simulink model "SrmAmLinearApcMmk1"  (R2013b)
settings: Solver=ode45  StartTime=0.0  StopTime=10.0  RelTol=1e-3
settings Model: Creator=mamingkai  LastModifiedBy=mamingkai

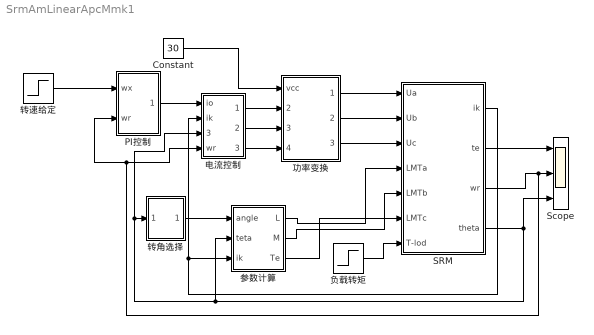
== system SrmAmLinearApcMmk1 ==
  Constant : Constant  Value=30
  PI控制 : Subsystem
  SRM : Subsystem
  Scope : Scope  NumInputPorts=3
      settings: YMin=-5~-5~-5  YMax=5~5~5
  功率变换 : Subsystem
  参数计算 : Subsystem
  电流控制 : Subsystem
  负载转矩 : Step  SampleTime=0
  转角选择 : Subsystem
  转速给定 : Step  SampleTime=0
  wires:
  转速给定/1 -> PI控制/1(wx)
  电流控制/1(Out1) -> 功率变换/2(PUSEA)
  电流控制/2(Out2) -> 功率变换/3(PUDEB)
  电流控制/3(Out3) -> 功率变换/4(PUSEC)
  PI控制/1(Out1) -> 电流控制/1(io)
  Constant/1 -> 功率变换/1(vcc)
  功率变换/1(Out1) -> SRM/1(Ua)
  功率变换/2(Out2) -> SRM/2(Ub)
  功率变换/3(Out3) -> SRM/3(Uc)
  转角选择/1(Out1) -> 参数计算/1(angle)
  SRM/1(ik) -> 参数计算/3(ik), 电流控制/2(ik)
  SRM/3(wr) -> PI控制/2(wr), 电流控制/4(wr), Scope/2
  SRM/4(theta) -> Scope/3, 转角选择/1(In1), 电流控制/3(teta), 参数计算/2(teta)
  SRM/2(te) -> Scope/1
  参数计算/1(L) -> SRM/4(LMTa)
  参数计算/2(M) -> SRM/5(LMTb)
  参数计算/3(Te) -> SRM/6(LMTc)
  负载转矩/1 -> SRM/7(T-lod)

== system SrmAmLinearApcMmk1/PI控制 ==
  wx : Inport
  wr : Inport  Port=2
  Gain : Gain
  Gain1 : Gain
  Integrator : Integrator
  Saturation : Saturate
  netsum : Sum  Inputs=2  SaturateOnIntegerOverflow=on  InputSameDT=on  OutDataTypeStr=Inherit: Same as first input
  netsum1 : Sum  Inputs=+-  SaturateOnIntegerOverflow=on  InputSameDT=on  OutDataTypeStr=Inherit: Same as first input
  Out1 : Outport
  wires:
  wx/1 -> netsum1/1
  wr/1 -> netsum1/2
  netsum1/1 -> Gain/1, Gain1/1
  Gain1/1 -> Integrator/1
  Integrator/1 -> netsum/2
  Gain/1 -> netsum/1
  netsum/1 -> Saturation/1
  Saturation/1 -> Out1/1

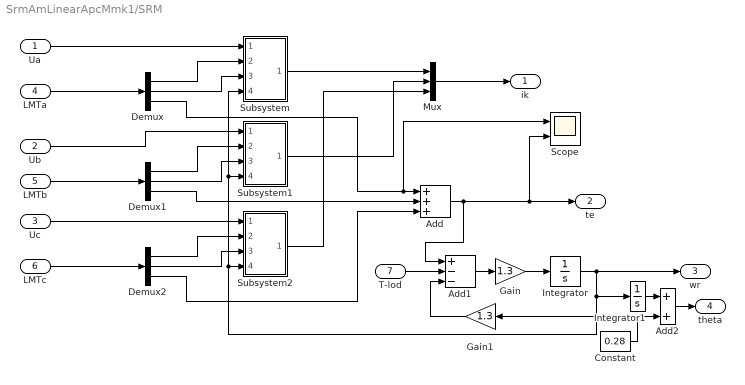
== system SrmAmLinearApcMmk1/SRM ==
  Ua : Inport
  Ub : Inport  Port=2
  Uc : Inport  Port=3
  LMTa : Inport  Port=4
  LMTb : Inport  Port=5
  LMTc : Inport  Port=6
  T-lod : Inport  Port=7
  Add : Sum  Inputs=+++
  Add1 : Sum  Inputs=+--
  Add2 : Sum
  Constant : Constant  Value=0.28
  Demux : Demux  Outputs=3
  Demux1 : Demux  Outputs=3
  Demux2 : Demux  Outputs=3
  Gain : Gain  Gain=1.3
  Gain1 : Gain  Gain=1.3
  Integrator : Integrator
  Integrator1 : Integrator
  Mux : Mux  Inputs=3
  Scope : Scope  NumInputPorts=2
      settings: YMin=-5~-5  YMax=5~5
  Subsystem : Subsystem
  Subsystem1 : Subsystem
  Subsystem2 : Subsystem
  ik : Outport
  te : Outport  Port=2
  wr : Outport  Port=3
  theta : Outport  Port=4
  wires:
  LMTa/1 -> Demux/1
  Demux/1 -> Subsystem/2(In2)
  Demux/2 -> Subsystem/3(In3)
  Demux/3 -> Scope/1, Add/1
  Ub/1 -> Subsystem1/1(In1)
  Demux1/1 -> Subsystem1/2(In2)
  Demux1/2 -> Subsystem1/3(In3)
  Demux1/3 -> Add/2
  Uc/1 -> Subsystem2/1(In1)
  LMTc/1 -> Demux2/1
  LMTb/1 -> Demux1/1
  Demux2/1 -> Subsystem2/2(In2)
  Demux2/2 -> Subsystem2/3(In3)
  Demux2/3 -> Add/3
  Integrator/1 -> wr/1, Subsystem2/4(In4), Subsystem1/4(In4), Subsystem/4(In4), Gain1/1, Integrator1/1
  Subsystem/1(Out1) -> Mux/1
  Subsystem1/1(Out1) -> Mux/2
  Subsystem2/1(Out1) -> Mux/3
  Mux/1 -> ik/1
  Add/1 -> te/1, Scope/2, Add1/1
  T-lod/1 -> Add1/2
  Gain1/1 -> Add1/3
  Add1/1 -> Gain/1
  Gain/1 -> Integrator/1
  Add2/1 -> theta/1
  Integrator1/1 -> Add2/1
  Constant/1 -> Add2/2
  Ua/1 -> Subsystem/1(In1)

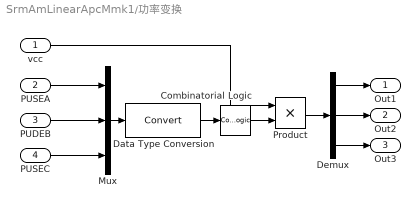
== system SrmAmLinearApcMmk1/功率变换 ==
  vcc : Inport
  PUSEA : Inport  Port=2
  PUDEB : Inport  Port=3
  PUSEC : Inport  Port=4
  Combinatorial Logic : CombinatorialLogic
  Data Type Conversion : DataTypeConversion
  Demux : Demux  Outputs=3
  Mux : Mux  Inputs=3
  Product : Product
  Out1 : Outport
  Out2 : Outport  Port=2
  Out3 : Outport  Port=3
  wires:
  PUSEA/1 -> Mux/1
  Demux/1 -> Out1/1
  Product/1 -> Demux/1
  Demux/2 -> Out2/1
  Demux/3 -> Out3/1
  PUDEB/1 -> Mux/2
  PUSEC/1 -> Mux/3
  Combinatorial Logic/1 -> Product/2
  vcc/1 -> Product/1
  Mux/1 -> Data Type Conversion/1
  Data Type Conversion/1 -> Combinatorial Logic/1

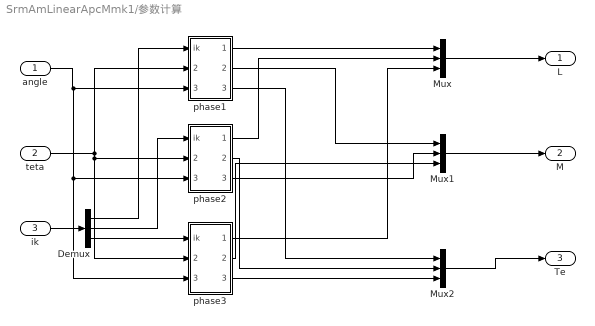
== system SrmAmLinearApcMmk1/参数计算 ==
  angle : Inport
  teta : Inport  Port=2
  ik : Inport  Port=3
  Demux : Demux  Outputs=3
  Mux : Mux  Inputs=3
  Mux1 : Mux  Inputs=3
  Mux2 : Mux  Inputs=3
  phase1 : Subsystem
  phase2 : Subsystem
  phase3 : Subsystem
  L : Outport
  M : Outport  Port=2
  Te : Outport  Port=3
  wires:
  teta/1 -> phase2/2(teta), phase3/2(teta), phase1/2(teta)
  Mux/1 -> L/1
  angle/1 -> phase2/3(angle), phase3/3(angle), phase1/3(angle)
  ik/1 -> Demux/1
  Demux/1 -> phase1/1(ik)
  Demux/2 -> phase2/1(ik)
  Demux/3 -> phase3/1(ik)
  phase1/1(Out1) -> Mux/1
  phase1/2(Out2) -> Mux1/1
  phase1/3(Out3) -> Mux2/1
  phase2/1(Out1) -> Mux/2
  phase2/3(Out3) -> Mux1/2
  phase2/2(Out2) -> Mux2/2
  phase3/1(Out1) -> Mux/3
  phase3/2(Out2) -> Mux1/3
  phase3/3(Out3) -> Mux2/3
  Mux1/1 -> M/1
  Mux2/1 -> Te/1

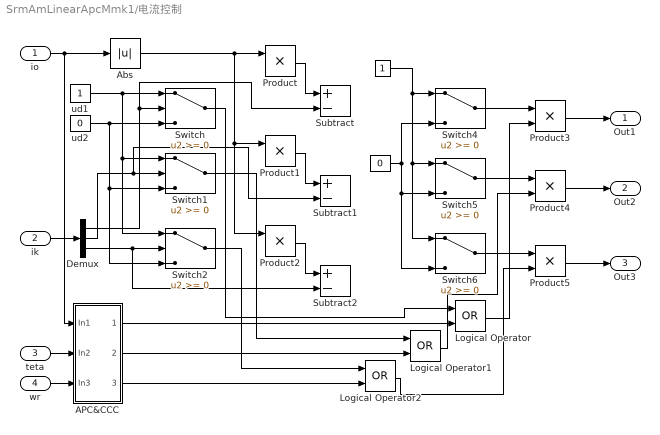
== system SrmAmLinearApcMmk1/电流控制 ==
  io : Inport
  ik : Inport  Port=2
  teta : Inport  Port=3
  wr : Inport  Port=4
  " " : Constant
  " " : Constant  Value=0
  APC&CCC : Subsystem
  Abs : Abs
  Demux : Demux  Outputs=3
  Logical Operator : Logic  Operator=OR  AllPortsSameDT=off  OutDataTypeStr=boolean
  Logical Operator1 : Logic  Operator=OR  AllPortsSameDT=off  OutDataTypeStr=boolean
  Logical Operator2 : Logic  Operator=OR  AllPortsSameDT=off  OutDataTypeStr=boolean
  Product{,1..5} (6 alike) : Product
  Subtract : Sum  Inputs=+-
  Subtract1 : Sum  Inputs=+-
  Subtract2 : Sum  Inputs=+-
  Switch{,1..2,4..6} (6 alike) : Switch
  ud1 : Constant
  ud2 : Constant  Value=0
  Out1 : Outport
  Out2 : Outport  Port=2
  Out3 : Outport  Port=3
  wires:
  ik/1 -> Demux/1
  io/1 -> APC&CCC/1(In1), Abs/1
  Abs/1 -> Product2/1, Product1/1, Product/1
  ud1/1 -> Switch2/1, Switch1/1, Switch/1
  ud2/1 -> Switch2/3, Switch1/3, Switch/3
  teta/1 -> APC&CCC/2(In2)
  Demux/1 -> Subtract/2, Switch/2
  Demux/3 -> Subtract2/2, Switch2/2
  Demux/2 -> Subtract1/2, Switch1/2
  APC&CCC/1(Out1) -> Logical Operator/2
  APC&CCC/2(Out2) -> Logical Operator1/2
  APC&CCC/3(Out3) -> Logical Operator2/2
  Switch/1 -> Logical Operator/1
  Switch1/1 -> Logical Operator1/1
  Switch2/1 -> Logical Operator2/1
  Product/1 -> Subtract/1
  Product1/1 -> Subtract1/1
  Product2/1 -> Subtract2/1
  " "/1 -> Switch6/1, Switch5/1, Switch4/1
  " "/1 -> Switch6/3, Switch5/3, Switch4/3
  wr/1 -> APC&CCC/3(In3)
  Logical Operator/1 -> Product3/2
  Logical Operator1/1 -> Product4/2
  Logical Operator2/1 -> Product5/2
  Switch6/1 -> Product5/1
  Switch5/1 -> Product4/1
  Switch4/1 -> Product3/1
  Product3/1 -> Out1/1
  Product4/1 -> Out2/1
  Product5/1 -> Out3/1

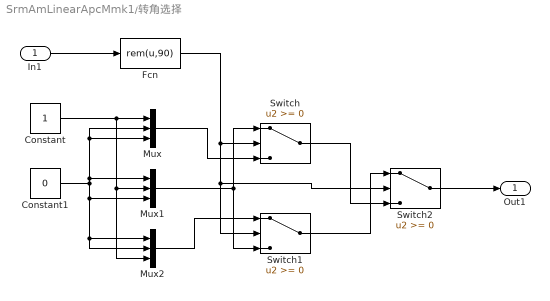
== system SrmAmLinearApcMmk1/转角选择 ==
  In1 : Inport
  Constant : Constant
  Constant1 : Constant  Value=0
  Fcn : Fcn  Expr=rem(u,90)
  Mux : Mux  Inputs=3
  Mux1 : Mux  Inputs=3
  Mux2 : Mux  Inputs=3
  Switch : Switch
  Switch1 : Switch
  Switch2 : Switch
  Out1 : Outport
  wires:
  In1/1 -> Fcn/1
  Constant/1 -> Mux2/3, Mux1/2, Mux/1
  Mux/1 -> Switch/3
  Constant1/1 -> Mux1/1, Mux/3, Mux/2, Mux2/2, Mux2/1, Mux1/3
  Mux1/1 -> Switch/1, Switch1/3
  Mux2/1 -> Switch1/1
  Fcn/1 -> Switch2/2, Switch1/2, Switch/2
  Switch/1 -> Switch2/3
  Switch1/1 -> Switch2/1
  Switch2/1 -> Out1/1

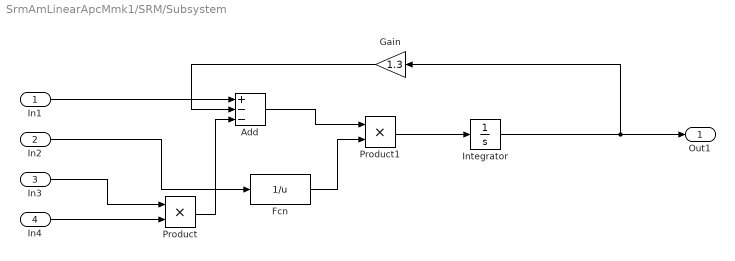
== system SrmAmLinearApcMmk1/SRM/Subsystem ==
  In1 : Inport
  In2 : Inport  Port=2
  In3 : Inport  Port=3
  In4 : Inport  Port=4
  Add : Sum  Inputs=+--
  Fcn : Fcn  Expr=1/u
  Gain : Gain  Gain=1.3
  Integrator : Integrator
  Product : Product
  Product1 : Product
  Out1 : Outport
  wires:
  In4/1 -> Product/2
  Integrator/1 -> Gain/1, Out1/1
  In3/1 -> Product/1
  In2/1 -> Fcn/1
  In1/1 -> Add/1
  Gain/1 -> Add/2
  Product/1 -> Add/3
  Add/1 -> Product1/1
  Fcn/1 -> Product1/2
  Product1/1 -> Integrator/1

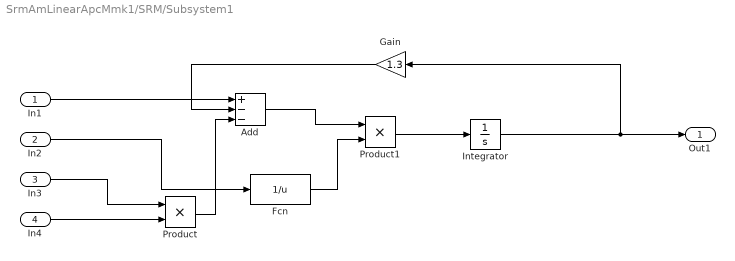
== system SrmAmLinearApcMmk1/SRM/Subsystem1 ==
  In1 : Inport
  In2 : Inport  Port=2
  In3 : Inport  Port=3
  In4 : Inport  Port=4
  Add : Sum  Inputs=+--
  Fcn : Fcn  Expr=1/u
  Gain : Gain  Gain=1.3
  Integrator : Integrator
  Product : Product
  Product1 : Product
  Out1 : Outport
  wires:
  In4/1 -> Product/2
  Integrator/1 -> Gain/1, Out1/1
  In3/1 -> Product/1
  In2/1 -> Fcn/1
  In1/1 -> Add/1
  Gain/1 -> Add/2
  Product/1 -> Add/3
  Add/1 -> Product1/1
  Fcn/1 -> Product1/2
  Product1/1 -> Integrator/1

== system SrmAmLinearApcMmk1/SRM/Subsystem2 ==
  In1 : Inport
  In2 : Inport  Port=2
  In3 : Inport  Port=3
  In4 : Inport  Port=4
  Add : Sum  Inputs=+--
  Fcn : Fcn  Expr=1/u
  Gain : Gain  Gain=1.3
  Integrator : Integrator
  Product : Product
  Product1 : Product
  Out1 : Outport
  wires:
  In4/1 -> Product/2
  Integrator/1 -> Gain/1, Out1/1
  In3/1 -> Product/1
  In2/1 -> Fcn/1
  In1/1 -> Add/1
  Gain/1 -> Add/2
  Product/1 -> Add/3
  Add/1 -> Product1/1
  Fcn/1 -> Product1/2
  Product1/1 -> Integrator/1

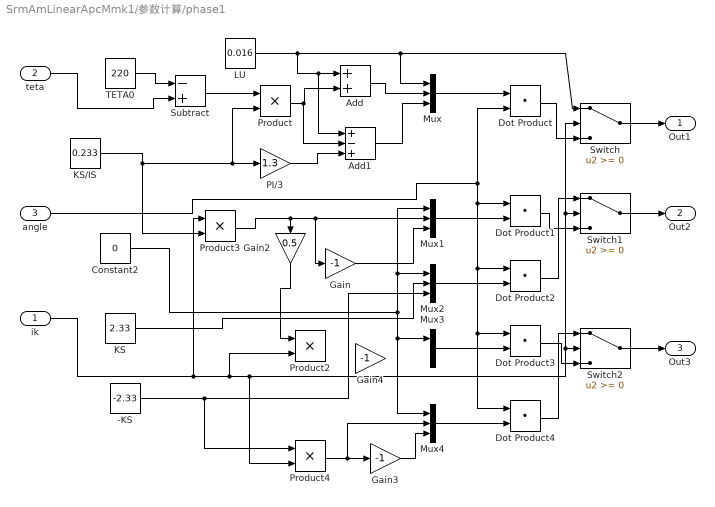
== system SrmAmLinearApcMmk1/参数计算/phase1 ==
  ik : Inport
  teta : Inport  Port=2
  angle : Inport  Port=3
  -KS : Constant  Value=-2.33
  Add : Sum
  Add1 : Sum  Inputs=+-+
  Constant2 : Constant  Value=0
  Dot Product{,1..4} (5 alike) : DotProduct  InputSameDT=on  OutDataTypeStr=Inherit: Inherit via internal rule
  Gain : Gain  Gain=-1
  Gain2 : Gain  Gain=0.5
  Gain3 : Gain  Gain=-1
  Gain4 : Gain  Gain=-1
  KS : Constant  Value=2.33
  KS/IS : Constant  Value=0.233
  LU : Constant  Value=0.016
  Mux{,1..4} (5 alike) : Mux  Inputs=3
  PI/3 : Gain  Gain=1.3
  Product{,2..4} (4 alike) : Product
  Subtract : Sum  Inputs=-+
  Switch : Switch
  Switch1 : Switch
  Switch2 : Switch
  TETA0 : Constant  Value=220
  Out1 : Outport
  Out2 : Outport  Port=2
  Out3 : Outport  Port=3
  wires:
  Switch/1 -> Out1/1
  teta/1 -> Subtract/2
  TETA0/1 -> Subtract/1
  Subtract/1 -> Product/1
  KS/IS/1 -> PI/3/1, Product/2, Product3/2
  LU/1 -> Switch/1, Mux/1, Add1/1, Add/1
  Product/1 -> Add1/2, Add/2
  PI/3/1 -> Add1/3
  Add/1 -> Mux/2
  Add1/1 -> Mux/3
  Mux/1 -> Dot Product/1
  Dot Product/1 -> Switch/3
  ik/1 -> Product3/1, Product2/2, Product4/2, Switch2/2, Switch1/2, Switch/2
  angle/1 -> Dot Product4/1, Dot Product3/1, Dot Product2/1, Dot Product1/1, Dot Product/2
  Mux4/1 -> Dot Product4/2
  Constant2/1 -> Mux4/1, Mux3/1, Mux2/1, Mux1/1
  Mux3/1 -> Dot Product3/2
  Mux2/1 -> Dot Product2/2
  Mux1/1 -> Dot Product1/2
  KS/1 -> Mux2/2
  -KS/1 -> Product4/1, Mux2/3
  Product3/1 -> Gain2/1, Gain/1, Mux1/2
  Gain/1 -> Mux1/3
  Gain2/1 -> Product2/1
  Product4/1 -> Gain3/1, Mux4/2
  Gain3/1 -> Mux4/3
  Dot Product4/1 -> Switch2/1
  Dot Product3/1 -> Switch2/3
  Dot Product2/1 -> Switch1/1
  Dot Product1/1 -> Switch1/3
  Switch1/1 -> Out2/1
  Switch2/1 -> Out3/1

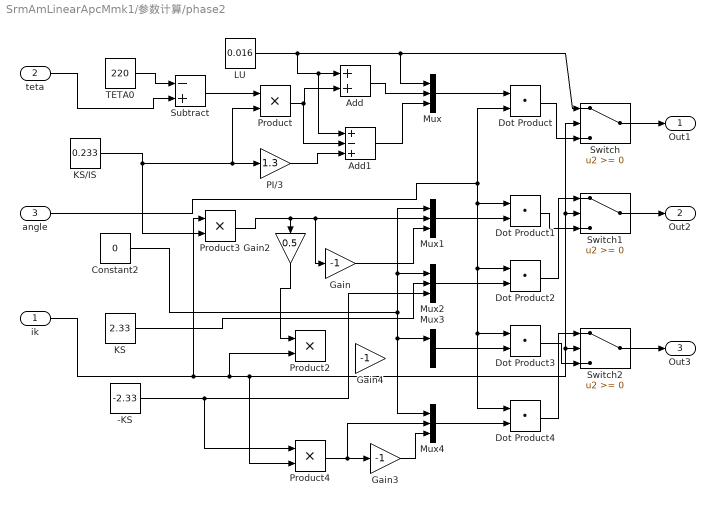
== system SrmAmLinearApcMmk1/参数计算/phase2 ==
  ik : Inport
  teta : Inport  Port=2
  angle : Inport  Port=3
  -KS : Constant  Value=-2.33
  Add : Sum
  Add1 : Sum  Inputs=+-+
  Constant2 : Constant  Value=0
  Dot Product{,1..4} (5 alike) : DotProduct  InputSameDT=on  OutDataTypeStr=Inherit: Inherit via internal rule
  Gain : Gain  Gain=-1
  Gain2 : Gain  Gain=0.5
  Gain3 : Gain  Gain=-1
  Gain4 : Gain  Gain=-1
  KS : Constant  Value=2.33
  KS/IS : Constant  Value=0.233
  LU : Constant  Value=0.016
  Mux{,1..4} (5 alike) : Mux  Inputs=3
  PI/3 : Gain  Gain=1.3
  Product{,2..4} (4 alike) : Product
  Subtract : Sum  Inputs=-+
  Switch : Switch
  Switch1 : Switch
  Switch2 : Switch
  TETA0 : Constant  Value=220
  Out1 : Outport
  Out2 : Outport  Port=2
  Out3 : Outport  Port=3
  wires:
  Switch/1 -> Out1/1
  teta/1 -> Subtract/2
  TETA0/1 -> Subtract/1
  Subtract/1 -> Product/1
  KS/IS/1 -> PI/3/1, Product/2, Product3/2
  LU/1 -> Switch/1, Mux/1, Add1/1, Add/1
  Product/1 -> Add1/2, Add/2
  PI/3/1 -> Add1/3
  Add/1 -> Mux/2
  Add1/1 -> Mux/3
  Mux/1 -> Dot Product/1
  Dot Product/1 -> Switch/3
  ik/1 -> Product3/1, Product2/2, Product4/2, Switch2/2, Switch1/2, Switch/2
  angle/1 -> Dot Product4/1, Dot Product3/1, Dot Product2/1, Dot Product1/1, Dot Product/2
  Mux4/1 -> Dot Product4/2
  Constant2/1 -> Mux4/1, Mux3/1, Mux2/1, Mux1/1
  Mux3/1 -> Dot Product3/2
  Mux2/1 -> Dot Product2/2
  Mux1/1 -> Dot Product1/2
  KS/1 -> Mux2/2
  -KS/1 -> Product4/1, Mux2/3
  Product3/1 -> Gain2/1, Gain/1, Mux1/2
  Gain/1 -> Mux1/3
  Gain2/1 -> Product2/1
  Product4/1 -> Gain3/1, Mux4/2
  Gain3/1 -> Mux4/3
  Dot Product4/1 -> Switch2/1
  Dot Product3/1 -> Switch2/3
  Dot Product2/1 -> Switch1/1
  Dot Product1/1 -> Switch1/3
  Switch1/1 -> Out2/1
  Switch2/1 -> Out3/1

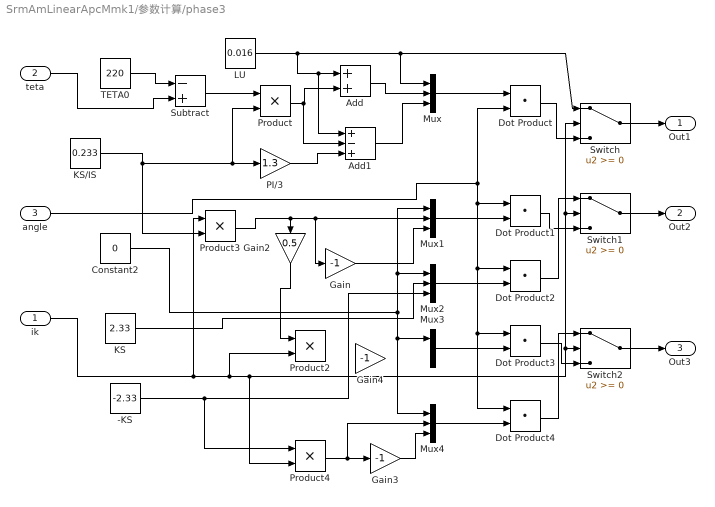
== system SrmAmLinearApcMmk1/参数计算/phase3 ==
  ik : Inport
  teta : Inport  Port=2
  angle : Inport  Port=3
  -KS : Constant  Value=-2.33
  Add : Sum
  Add1 : Sum  Inputs=+-+
  Constant2 : Constant  Value=0
  Dot Product{,1..4} (5 alike) : DotProduct  InputSameDT=on  OutDataTypeStr=Inherit: Inherit via internal rule
  Gain : Gain  Gain=-1
  Gain2 : Gain  Gain=0.5
  Gain3 : Gain  Gain=-1
  Gain4 : Gain  Gain=-1
  KS : Constant  Value=2.33
  KS/IS : Constant  Value=0.233
  LU : Constant  Value=0.016
  Mux{,1..4} (5 alike) : Mux  Inputs=3
  PI/3 : Gain  Gain=1.3
  Product{,2..4} (4 alike) : Product
  Subtract : Sum  Inputs=-+
  Switch : Switch
  Switch1 : Switch
  Switch2 : Switch
  TETA0 : Constant  Value=220
  Out1 : Outport
  Out2 : Outport  Port=2
  Out3 : Outport  Port=3
  wires:
  Switch/1 -> Out1/1
  teta/1 -> Subtract/2
  TETA0/1 -> Subtract/1
  Subtract/1 -> Product/1
  KS/IS/1 -> PI/3/1, Product/2, Product3/2
  LU/1 -> Switch/1, Mux/1, Add1/1, Add/1
  Product/1 -> Add1/2, Add/2
  PI/3/1 -> Add1/3
  Add/1 -> Mux/2
  Add1/1 -> Mux/3
  Mux/1 -> Dot Product/1
  Dot Product/1 -> Switch/3
  ik/1 -> Product3/1, Product2/2, Product4/2, Switch2/2, Switch1/2, Switch/2
  angle/1 -> Dot Product4/1, Dot Product3/1, Dot Product2/1, Dot Product1/1, Dot Product/2
  Mux4/1 -> Dot Product4/2
  Constant2/1 -> Mux4/1, Mux3/1, Mux2/1, Mux1/1
  Mux3/1 -> Dot Product3/2
  Mux2/1 -> Dot Product2/2
  Mux1/1 -> Dot Product1/2
  KS/1 -> Mux2/2
  -KS/1 -> Product4/1, Mux2/3
  Product3/1 -> Gain2/1, Gain/1, Mux1/2
  Gain/1 -> Mux1/3
  Gain2/1 -> Product2/1
  Product4/1 -> Gain3/1, Mux4/2
  Gain3/1 -> Mux4/3
  Dot Product4/1 -> Switch2/1
  Dot Product3/1 -> Switch2/3
  Dot Product2/1 -> Switch1/1
  Dot Product1/1 -> Switch1/3
  Switch1/1 -> Out2/1
  Switch2/1 -> Out3/1

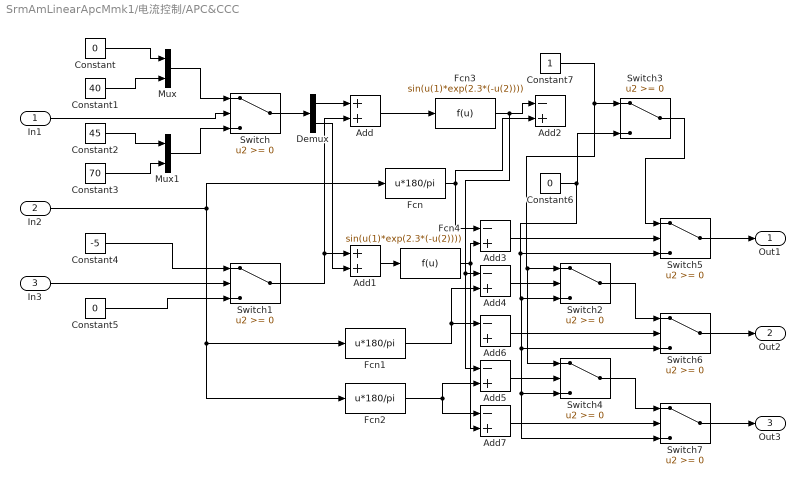
== system SrmAmLinearApcMmk1/电流控制/APC&CCC ==
  In1 : Inport
  In2 : Inport  Port=2
  In3 : Inport  Port=3
  Add : Sum
  Add1 : Sum
  Add{2..7} (6 alike) : Sum  Inputs=-+
  Constant : Constant  Value=0
  Constant1 : Constant  Value=40
  Constant2 : Constant  Value=45
  Constant3 : Constant  Value=70
  Constant4 : Constant  Value=-5
  Constant5 : Constant  Value=0
  Constant6 : Constant  Value=0
  Constant7 : Constant
  Demux : Demux  Outputs=2
  Fcn : Fcn  Expr=u*180/pi
  Fcn1 : Fcn  Expr=u*180/pi
  Fcn2 : Fcn  Expr=u*180/pi
  Fcn3 : Fcn  Expr=sin(u(1)*exp(2.3*(-u(2))))
  Fcn4 : Fcn  Expr=sin(u(1)*exp(2.3*(-u(2))))
  Mux : Mux  Inputs=2
  Mux1 : Mux  Inputs=2
  Switch{,1..7} (8 alike) : Switch
  Out1 : Outport
  Out2 : Outport  Port=2
  Out3 : Outport  Port=3
  wires:
  Switch5/1 -> Out1/1
  In3/1 -> Switch1/2
  In1/1 -> Switch/2
  In2/1 -> Fcn/1, Fcn2/1, Fcn1/1
  Mux/1 -> Switch/1
  Constant4/1 -> Switch1/1
  Constant5/1 -> Switch1/3
  Constant/1 -> Mux/1
  Constant1/1 -> Mux/2
  Constant2/1 -> Mux1/1
  Constant3/1 -> Mux1/2
  Mux1/1 -> Switch/3
  Switch/1 -> Demux/1
  Demux/1 -> Add/1
  Demux/2 -> Add1/2
  Switch1/1 -> Add1/1, Add/2
  Add1/1 -> Fcn4/1
  Fcn4/1 -> Add3/2, Add7/2
  Add/1 -> Fcn3/1
  Fcn3/1 -> Add5/1, Add4/1, Add2/1
  Fcn/1 -> Add2/2, Add3/1
  Fcn1/1 -> Add6/1, Add4/2
  Fcn2/1 -> Add7/1, Add5/2
  Add3/1 -> Switch5/2
  Add4/1 -> Switch2/2
  Add6/1 -> Switch6/2
  Add5/1 -> Switch4/2
  Add7/1 -> Switch7/2
  Constant7/1 -> Switch4/1, Switch2/1, Switch3/1
  Constant6/1 -> Switch6/3, Switch7/3, Switch4/3, Switch2/3, Switch5/3, Switch3/3
  Switch3/1 -> Switch5/1
  Switch2/1 -> Switch6/1
  Switch4/1 -> Switch7/1
  Switch6/1 -> Out2/1
  Switch7/1 -> Out3/1
